simulink model "Lab_model_EOM"  (R2025b)
settings: Solver=VariableStepAuto  StartTime=0.0  StopTime=t_stop  RelTol=1e-3
undefined symbols (not defined in the file): c1, c2, c3, c4, init_chassis, init_seat, init_wheel, k1, k2, k3, m1, m2, m3
settings Model: Creator=LEGION  LastModifiedBy=LEGION
settings DataIOCC: ReturnWorkspaceOutputs=off

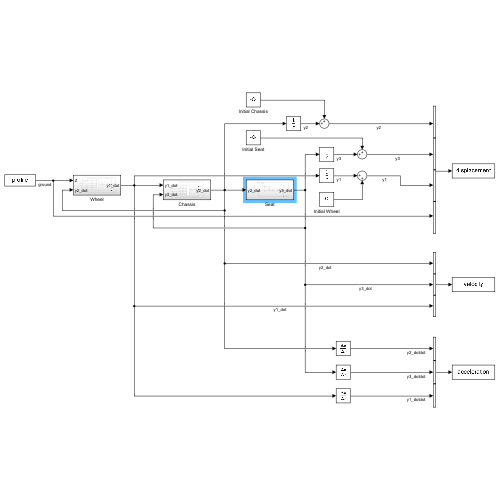
[thumbnail: Simulink's stored preview of the top-level diagram]
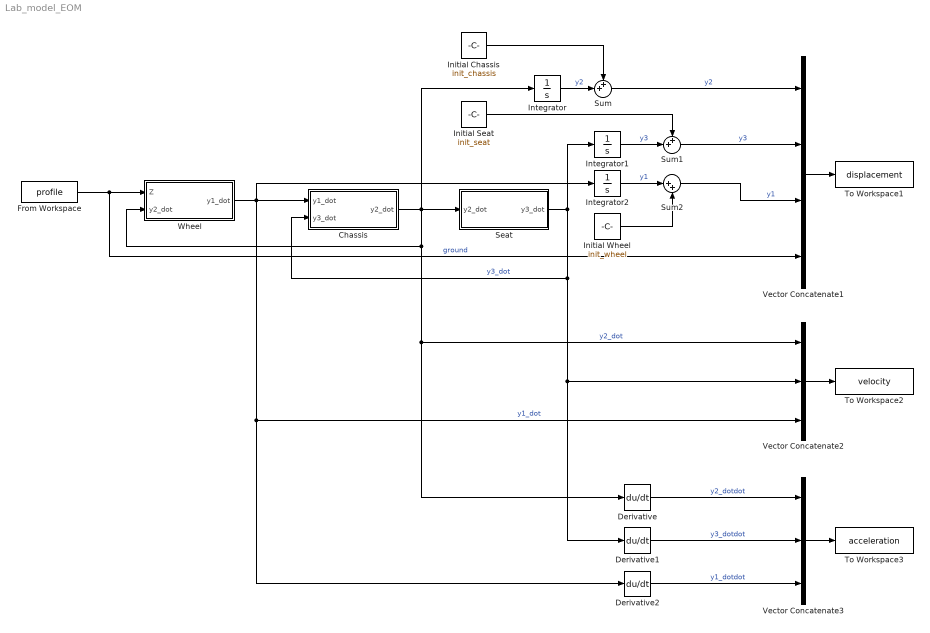
== system Lab_model_EOM ==
  Chassis : Subsystem
  Derivative : Derivative
  Derivative1 : Derivative
  Derivative2 : Derivative
  From Workspace : FromWorkspace  VariableName=profile
  Initial Chassis : Constant  Value=init_chassis
  Initial Seat : Constant  Value=init_seat
  Initial Wheel : Constant  Value=init_wheel
  Integrator : Integrator
  Integrator1 : Integrator
  Integrator2 : Integrator
  Seat : Subsystem
  Sum : Sum  Inputs=++|
  Sum1 : Sum  Inputs=++|
  Sum2 : Sum  Inputs=|++
  To Workspace1 : ToWorkspace  VariableName=displacement  SaveFormat=Structure With Time  SampleTime=-1
  To Workspace2 : ToWorkspace  VariableName=velocity  SaveFormat=Structure With Time  SampleTime=-1
  To Workspace3 : ToWorkspace  VariableName=acceleration  SaveFormat=Structure With Time  SampleTime=-1
  Vector Concatenate1 : Concatenate  NumInputs=4
  Vector Concatenate2 : Concatenate  NumInputs=3
  Vector Concatenate3 : Concatenate  NumInputs=3
  Wheel : Subsystem
  wires:
  Chassis/1(y2_dot) -> Integrator/1, Derivative/1, Vector Concatenate2/1, Wheel/2(y2_dot), Seat/1(y2_dot)  "y2_dot"
  Wheel/1(y1_dot) -> Derivative2/1, Vector Concatenate2/3, Integrator2/1, Chassis/1(y1_dot)  "y1_dot"
  Seat/1(y3_dot) -> Integrator1/1, Chassis/2(y3_dot), Derivative1/1, Vector Concatenate2/2  "y3_dot"
  From Workspace/1 -> Vector Concatenate1/4, Wheel/1(Z)  "ground"
  Initial Chassis/1 -> Sum/1
  Integrator/1 -> Sum/2  "y2"
  Sum/1 -> Vector Concatenate1/1  "y2"
  Initial Seat/1 -> Sum1/1
  Integrator1/1 -> Sum1/2  "y3"
  Sum1/1 -> Vector Concatenate1/2  "y3"
  Sum2/1 -> Vector Concatenate1/3  "y1"
  Integrator2/1 -> Sum2/1  "y1"
  Initial Wheel/1 -> Sum2/2
  Derivative1/1 -> Vector Concatenate3/2  "y3_dotdot"
  Derivative/1 -> Vector Concatenate3/1  "y2_dotdot"
  Derivative2/1 -> Vector Concatenate3/3  "y1_dotdot"
  Vector Concatenate1/1 -> To Workspace1/1
  Vector Concatenate3/1 -> To Workspace3/1
  Vector Concatenate2/1 -> To Workspace2/1

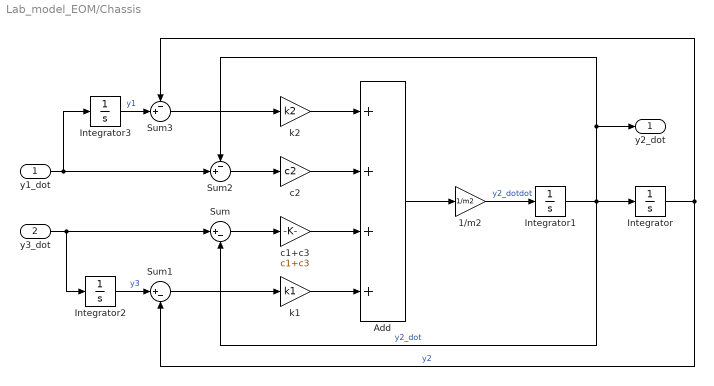
== system Lab_model_EOM/Chassis ==
  y1_dot : Inport
  y3_dot : Inport  Port=2
  1/m2 : Gain  Gain=1/m2
  Add : Sum  Inputs=++++
  Integrator{,1..3} (4 alike) : Integrator
  Sum : Sum  Inputs=|+-
  Sum1 : Sum  Inputs=|+-
  Sum2 : Sum  Inputs=-+|
  Sum3 : Sum  Inputs=-+|
  c1+c3 : Gain  Gain=c1+c3
  c2 : Gain  Gain=c2
  k1 : Gain  Gain=k1
  k2 : Gain  Gain=k2
  y2_dot : Outport
  wires:
  1/m2/1 -> Integrator1/1  "y2_dotdot"
  Integrator1/1 -> Integrator/1, y2_dot/1, Sum2/1, Sum/2  "y2_dot"
  Integrator/1 -> Sum3/1, Sum1/2  "y2"
  y3_dot/1 -> Sum/1, Integrator2/1
  Sum/1 -> c1+c3/1
  c1+c3/1 -> Add/3
  Integrator2/1 -> Sum1/1  "y3"
  Sum1/1 -> k1/1
  k1/1 -> Add/4
  Add/1 -> 1/m2/1
  y1_dot/1 -> Integrator3/1, Sum2/2
  Sum2/1 -> c2/1
  c2/1 -> Add/2
  Integrator3/1 -> Sum3/2  "y1"
  Sum3/1 -> k2/1
  k2/1 -> Add/1

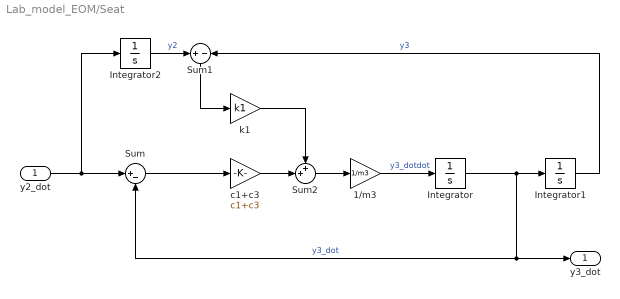
== system Lab_model_EOM/Seat ==
  y2_dot : Inport
  1/m3 : Gain  Gain=1/m3
  Integrator : Integrator
  Integrator1 : Integrator
  Integrator2 : Integrator
  Sum : Sum  Inputs=|+-
  Sum1 : Sum  Inputs=+|-
  Sum2 : Sum  Inputs=++|
  c1+c3 : Gain  Gain=c1+c3
  k1 : Gain  Gain=k1
  y3_dot : Outport
  wires:
  y2_dot/1 -> Integrator2/1, Sum/1
  1/m3/1 -> Integrator/1  "y3_dotdot"
  Integrator/1 -> y3_dot/1, Sum/2, Integrator1/1  "y3_dot"
  Integrator1/1 -> Sum1/2  "y3"
  Sum/1 -> c1+c3/1
  Integrator2/1 -> Sum1/1  "y2"
  Sum1/1 -> k1/1
  c1+c3/1 -> Sum2/2
  k1/1 -> Sum2/1
  Sum2/1 -> 1/m3/1

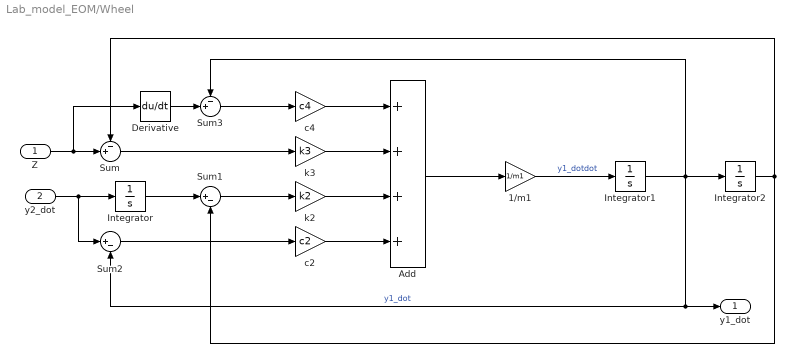
== system Lab_model_EOM/Wheel ==
  Z : Inport
  y2_dot : Inport  Port=2
  1/m1 : Gain  Gain=1/m1
  Add : Sum  Inputs=++++
  Derivative : Derivative
  Integrator : Integrator
  Integrator1 : Integrator
  Integrator2 : Integrator
  Sum : Sum  Inputs=-+|
  Sum1 : Sum  Inputs=|+-
  Sum2 : Sum  Inputs=|+-
  Sum3 : Sum  Inputs=-+|
  c2 : Gain  Gain=c2
  c4 : Gain  Gain=c4
  k2 : Gain  Gain=k2
  k3 : Gain  Gain=k3
  y1_dot : Outport
  wires:
  y2_dot/1 -> Sum2/1, Integrator/1
  Add/1 -> 1/m1/1
  1/m1/1 -> Integrator1/1  "y1_dotdot"
  Integrator1/1 -> Sum3/1, Sum2/2, y1_dot/1, Integrator2/1  "y1_dot"
  Integrator2/1 -> Sum1/2, Sum/1
  Z/1 -> Derivative/1, Sum/2
  Sum/1 -> k3/1
  Integrator/1 -> Sum1/1
  Sum1/1 -> k2/1
  Sum2/1 -> c2/1
  c2/1 -> Add/4
  k2/1 -> Add/3
  k3/1 -> Add/2
  Derivative/1 -> Sum3/2
  Sum3/1 -> c4/1
  c4/1 -> Add/1
